simulink library "sltestProjectorCtrlAssessLibrary"  (R2018a)
settings: Solver=ode45  StartTime=0.0  StopTime=10.0  RelTol=1e-3  EnableMultiTasking=on
settings Model: Creator=The MathWorks, Inc.  LastModifiedBy=The MathWorks, Inc.
settings DataIOCC: LimitDataPoints=on  SaveFormat=Array
settings OptimizationCC: LifeSpan=inf
settings DebuggingCC: SolverPrmCheckMsg=warning  AllowSymbolicDim=off  SFUnexpectedBacktrackingDiag=warning  SFNoUnconditionalDefaultTransitionDiag=warning  SFExecutionAtInitializationDiag=none
settings ModelReferenceCC: PropagateSignalLabelsOutOfModel=off
settings CodeAppCC: StateflowObjectComments=on
settings GRTTargetCC: TargetLangStandard=C89/C90 (ANSI)  GeneratePreprocessorConditionals=Disable all
settings ConfigComp: CovMetricSettings=dw  CovHtmlReporting=on  CovSaveCumulativeToWorkspaceVar=on  CovSaveSingleToWorkspaceVar=on  CovExternalEMLEnable=off  CovSFcnEnable=off

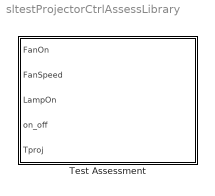
== system sltestProjectorCtrlAssessLibrary ==
  Test Assessment : Test Sequence  RequirementInfo="{}  %GIDa_9b7a8a3d_12da_4d50_8830_b6b1ccf7c03a"  TreatAsAtomicUnit=on

== stateflow chart sltestProjectorCtrlAssessLibrary/Test Assessment ==
  settings: stateMachineType=SIMPLIFIED_MACHINE
  state GlobalAssess
    verify(~LampOn == true || FanOn == true,...
    'Simulink:verify_lamp_implies_fan',...
    'Fan must be on if lamp is on');
    settings: description=|
        | The logical statement inside this
        | verify statement is equivalent to
        | LampOn -> FanOn. See
        | requirement 1.4.
    state OverheatCondition
      verify(LampOn == false &&...
      FanOn == true && FanSpeed == High,...
      'Simulink:verify_overheat',...
      'In overheat condition lamp must be off and fan high');
    state HighTempCondition
      verify(FanOn == true && FanSpeed == High,...
      'Simulink:verify_high_temp',...
      'In high temp condition fan must be high');
    state NormalCondition
      verify(duration(FanSpeed == High) <= 10,...
      'Simulink:verify_fan_normal',...
      'In normal condition fan must return to normal within 10 s');
      settings: description=|
          | This verifies that the fan is never
          | at high for longer than 10 sec if
          | the projector is at a normal temp.
          | See requirement 1.8.
    state Else
    GlobalAssess -> (junction 22)
    (default) -> (junction 22)
    (junction 22) -> (junction 23) [order 1] : [Tproj > 65]
    (junction 23) -> OverheatCondition [order 1] : [~in(OverheatCondition)]
    (junction 22) -> (junction 31) [order 2]
    (junction 23) -> (junction 26) [order 2]
    (junction 31) -> (junction 32) [order 1] : [Tproj > 58]
    (junction 32) -> HighTempCondition [order 1] : [~in(HighTempCondition)]
    (junction 31) -> (junction 44) [order 2]
    (junction 32) -> (junction 35) [order 2]
    (junction 44) -> (junction 45) [order 1] : [(Tproj < 58 && LampOn == true)]
    (junction 45) -> NormalCondition [order 1] : [~in(NormalCondition)]
    (junction 45) -> (junction 48) [order 2]
    (junction 52) -> (junction 53)
    (junction 53) -> Else [order 1] : [~in(Else)]
    (junction 53) -> (junction 56) [order 2]
    (junction 44) -> (junction 52) [order 2]
  (default) -> GlobalAssess
  data: FanOn input boolean size=[1]; FanSpeed input Enum: FanSpeed size=[1]; LampOn input boolean size=[1]; on_off input boolean size=[1]; Tproj input single size=[1]
